simulink model "warplab_siso_unconverted_backup"  (Simulink 6.5)
settings: Solver=ode45  StartTime=0.0  StopTime=30000  RelTol=1e-3
libraries: xbsIndex_r4 x94, WARP_Blockset x4, simulink x1
settings Model: Creator=Melissa.Duarte  LastModifiedBy=cj.steuernagel
settings DebuggingCC: MultiTaskDSMMsg=warning  MultiTaskCondExecSysMsg=none
settings RTWCC: IncludeERTFirstTime=on

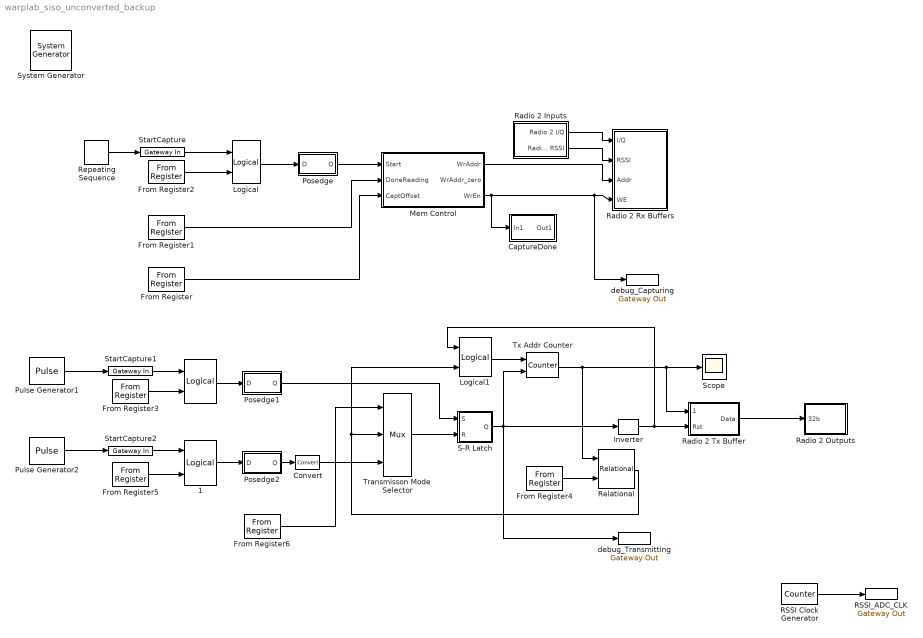
== system warplab_siso_unconverted_backup ==
  " " : xbsIndex_r4/Logical  logical_function=OR  inputs=2  en=off  latency=0  precision=Full  arith_type=Unsigned  n_bits=16  bin_pt=0  align_bp=on  dbl_ovrd=off  block_type=logical
      settings: block_version=9.1.01
  " 1" : xbsIndex_r4/Logical  logical_function=OR  inputs=2  en=off  latency=0  precision=Full  arith_type=Unsigned  n_bits=16  bin_pt=0  align_bp=on  dbl_ovrd=off  block_type=logical
      settings: block_version=9.1.01
  " System Generator" : xbsIndex_r4/ System Generator  Tag=genX  SystemSampleTime=-1  xilinxfamily=Virtex4  part=xc4vsx35  speed=-10  package=ff668  synthesis_tool=XST  directory=./netlist  testbench=off  simulink_period=1  sysclk_period=10  incr_netlist=off  trim_vbits=Everywhere in SubSystem  dbl_ovrd=According to Block Masks  core_generation=According to Block Masks  run_coregen=off  deprecated_control=off  eval_field=0  block_type=sysgen
      settings: block_version=8.2
  CaptureDone : Subsystem
  Convert : xbsIndex_r4/Convert  arith_type=Boolean  n_bits=16  bin_pt=14  quantization=Truncate  overflow=Wrap  latency=0  dbl_ovrd=off  pipeline=off  block_type=convert
  From Register : xbsIndex_r4/From Register  shared_memory_name='CaptOffset'  init=100  period=1  ownership=Locally owned and initialized  arith_type=Unsigned  n_bits=14  bin_pt=0  dbl_ovrd=off  block_type=fromreg
      settings: AttributesFormatString=CaptOffset\n<< %<shared_memory_name> >>  infoedit="Register block that reads data to a shared memory register.  Delay of one sample period."  block_version=8.2
  From Register1 : xbsIndex_r4/From Register  shared_memory_name='DoneReading'  init=0  period=1  ownership=Locally owned and initialized  arith_type=Unsigned  n_bits=1  bin_pt=0  dbl_ovrd=off  block_type=fromreg
      settings: AttributesFormatString=DoneReading\n<< %<shared_memory_name> >>  infoedit="Register block that reads data to a shared memory register.  Delay of one sample period."  block_version=8.2
  From Register2 : xbsIndex_r4/From Register  shared_memory_name='StartCapture'  init=0  period=1  ownership=Locally owned and initialized  arith_type=Unsigned  n_bits=1  bin_pt=0  dbl_ovrd=off  block_type=fromreg
      settings: AttributesFormatString=StartCapture\n<< %<shared_memory_name> >>  infoedit="Register block that reads data to a shared memory register.  Delay of one sample period."  block_version=8.2
  From Register3 : xbsIndex_r4/From Register  shared_memory_name='StartTx'  init=0  period=1  ownership=Locally owned and initialized  arith_type=Unsigned  n_bits=1  bin_pt=0  dbl_ovrd=off  block_type=fromreg
      settings: AttributesFormatString=StartTx\n<< %<shared_memory_name> >>  infoedit="Register block that reads data to a shared memory register.  Delay of one sample period."  block_version=8.2
  From Register4 : xbsIndex_r4/From Register  shared_memory_name='TxLength'  init=2^14-1  period=1  ownership=Locally owned and initialized  arith_type=Unsigned  n_bits=14  bin_pt=0  dbl_ovrd=off  block_type=fromreg
      settings: AttributesFormatString=TxLength\n<< %<shared_memory_name> >>  infoedit="Register block that reads data to a shared memory register.  Delay of one sample period."  block_version=8.2
  From Register5 : xbsIndex_r4/From Register  shared_memory_name='StopTx'  init=0  period=1  ownership=Locally owned and initialized  arith_type=Unsigned  n_bits=1  bin_pt=0  dbl_ovrd=off  block_type=fromreg
      settings: AttributesFormatString=StopTx\n<< %<shared_memory_name> >>  infoedit="Register block that reads data to a shared memory register.  Delay of one sample period."  block_version=8.2
  From Register6 : xbsIndex_r4/From Register  shared_memory_name='TransMode'  init=1  period=1  ownership=Locally owned and initialized  arith_type=Unsigned  n_bits=1  bin_pt=0  dbl_ovrd=off  block_type=fromreg
      settings: AttributesFormatString=TransMode\n<< %<shared_memory_name> >>  infoedit="Register block that reads data to a shared memory register.  Delay of one sample period."  block_version=8.2
  Inverter : xbsIndex_r4/Inverter  en=off  latency=0  dbl_ovrd=off  block_type=inv
      settings: block_version=8.2
  Logical : xbsIndex_r4/Logical  logical_function=OR  inputs=2  en=off  latency=0  precision=Full  arith_type=Unsigned  n_bits=16  bin_pt=0  align_bp=on  dbl_ovrd=off  block_type=logical
      settings: block_version=8.2
  Logical1 : xbsIndex_r4/Logical  logical_function=OR  inputs=2  en=off  latency=0  precision=Full  arith_type=Unsigned  n_bits=16  bin_pt=0  align_bp=on  dbl_ovrd=off  block_type=logical
      settings: block_version=9.1.01
  Mem Control : Subsystem
  Posedge : Subsystem
  Posedge1 : Subsystem
  Posedge2 : Subsystem
  Pulse Generator1 : DiscretePulseGenerator  Period=1000000  PulseWidth=50  PhaseDelay=2
  Pulse Generator2 : DiscretePulseGenerator  Period=1000000  PulseWidth=50  PhaseDelay=20000
  RSSI Clock Generator : xbsIndex_r4/Counter  cnt_type=Free Running  cnt_to=Inf  operation=Up  start_count=0  cnt_by_val=1  arith_type=Unsigned  n_bits=1  bin_pt=0  load_pin=off  rst=off  en=off  explicit_period=on  period=2  dbl_ovrd=off  use_behavioral_HDL=off  use_rpm=off  block_type=counter
      settings: block_version=VER_STRING_GOES_HERE
  RSSI_ADC_CLK : xbsIndex_r4/Gateway Out  hdl_port=on  timing_constraint=None  locs_specified=off  LOCs={}  block_type=gatewayout
      settings: infoedit="Gateway out block.  Converts Xilinx fixed point inputs into ouputs of type Simulink integer, double, or fixed point.<P><P>Hardware notes:  In hardware these blocks become top level output ports or are discarded, depending on how they are configured."  block_version=8.2
  Radio 2 Rx Buffers : Subsystem
  Radio 2 Tx Buffer : Subsystem
  Radio 2 Inputs : Subsystem
  Radio 2 Outputs : Subsystem
  Relational : xbsIndex_r4/Relational  mode=a>=b  en=off  latency=0  dbl_ovrd=off  block_type=relational
      settings: block_version=8.2
  Repeating Sequence : simulink/Sources/Repeating Sequence  SystemSampleTime=-1  rep_seq_t=[1 19999 20000 20001]  rep_seq_y=[0 0 1 0]
  S-R Latch : Subsystem
  Scope : Scope
      settings: YMin=0  YMax=17000  SaveName=ScopeData2
  StartCapture : xbsIndex_r4/Gateway In  arith_type=Unsigned  n_bits=1  bin_pt=0  quantization="Round  (unbiased: +/- Inf)"  overflow=Saturate  period=1  dbl_ovrd=off  timing_constraint=None  locs_specified=off  LOCs={}  block_type=gatewayin
      settings: infoedit="Gateway in block.  Converts inputs of type Simulink integer, double and fixed point to  Xilinx fixed point type.<P><P>Hardware notes:  In hardware these blocks become top level input ports."  block_version=VER_STRING_GOES_HERE
  StartCapture1 : xbsIndex_r4/Gateway In  arith_type=Unsigned  n_bits=1  bin_pt=0  quantization="Round  (unbiased: +/- Inf)"  overflow=Saturate  period=1  dbl_ovrd=off  timing_constraint=None  locs_specified=off  LOCs={}  block_type=gatewayin
      settings: infoedit="Gateway in block.  Converts inputs of type Simulink integer, double and fixed point to  Xilinx fixed point type.<P><P>Hardware notes:  In hardware these blocks become top level input ports."  block_version=VER_STRING_GOES_HERE
  StartCapture2 : xbsIndex_r4/Gateway In  arith_type=Unsigned  n_bits=1  bin_pt=0  quantization="Round  (unbiased: +/- Inf)"  overflow=Saturate  period=1  dbl_ovrd=off  timing_constraint=None  locs_specified=off  LOCs={}  block_type=gatewayin
      settings: infoedit="Gateway in block.  Converts inputs of type Simulink integer, double and fixed point to  Xilinx fixed point type.<P><P>Hardware notes:  In hardware these blocks become top level input ports."  block_version=VER_STRING_GOES_HERE
  Transmisson Mode Selector : xbsIndex_r4/Mux  inputs=2  en=off  latency=0  precision=Full  arith_type=Unsigned  n_bits=16  bin_pt=14  quantization=Truncate  overflow=Wrap  dbl_ovrd=off  block_type=mux
      settings: block_version=9.1.01
  Tx Addr Counter : xbsIndex_r4/Counter  cnt_type=Free Running  cnt_to=Inf  operation=Up  start_count=0  cnt_by_val=1  arith_type=Unsigned  n_bits=14  bin_pt=0  load_pin=off  rst=on  en=on  explicit_period=off  period=1  dbl_ovrd=off  use_behavioral_HDL=off  use_rpm=off  block_type=counter
      settings: block_version=8.2
  debug_Capturing : xbsIndex_r4/Gateway Out  hdl_port=on  timing_constraint=None  locs_specified=off  LOCs={}  block_type=gatewayout
      settings: infoedit="Gateway out block.  Converts Xilinx fixed point inputs into ouputs of type Simulink integer, double, or fixed point.<P><P>Hardware notes:  In hardware these blocks become top level output ports or are discarded, depending on how they are configured."  block_version=8.2
  debug_Transmitting : xbsIndex_r4/Gateway Out  hdl_port=on  timing_constraint=None  locs_specified=off  LOCs={}  block_type=gatewayout
      settings: infoedit="Gateway out block.  Converts Xilinx fixed point inputs into ouputs of type Simulink integer, double, or fixed point.<P><P>Hardware notes:  In hardware these blocks become top level output ports or are discarded, depending on how they are configured."  block_version=8.2
  wires:
  Posedge/1(Q) -> Mem Control/1(Start)
  Mem Control/3(WrEn) -> Radio 2 Rx Buffers/4(WE), debug_Capturing/1, CaptureDone/1(In1)
  Mem Control/1(WrAddr) -> Radio 2 Rx Buffers/3(Addr)
  From Register/1 -> Mem Control/3(CaptOffset)
  From Register1/1 -> Mem Control/2(DoneReading)
  Repeating Sequence/1 -> StartCapture/1
  From Register2/1 -> Logical/2
  Logical/1 -> Posedge/1(D)
  StartCapture/1 -> Logical/1
  Radio 2 Tx Buffer/1(Data) -> Radio 2 Outputs/1(32b)
  Tx Addr Counter/1 -> Relational/1, Radio 2 Tx Buffer/1(RdAddr), Scope/1
  S-R Latch/1(Q) -> Inverter/1, debug_Transmitting/1, Tx Addr Counter/2
  From Register4/1 -> Relational/2
  Inverter/1 -> Radio 2 Tx Buffer/2(Rst), Logical1/1
  Radio 2 Inputs/1(Radio 2 I/Q) -> Radio 2 Rx Buffers/1(I/Q)
  Radio 2 Inputs/2(Radio 2 RSSI) -> Radio 2 Rx Buffers/2(RSSI)
  RSSI Clock Generator/1 -> RSSI_ADC_CLK/1
  Posedge1/1(Q) -> S-R Latch/1(S)
  " "/1 -> Posedge1/1(D)
  From Register3/1 -> " "/2
  StartCapture1/1 -> " "/1
  " 1"/1 -> Posedge2/1(D)
  From Register5/1 -> " 1"/2
  StartCapture2/1 -> " 1"/1
  Relational/1 -> Transmisson Mode Selector/2, Logical1/2
  Logical1/1 -> Tx Addr Counter/1
  From Register6/1 -> Transmisson Mode Selector/1
  Transmisson Mode Selector/1 -> S-R Latch/2(R)
  Pulse Generator2/1 -> StartCapture2/1
  Pulse Generator1/1 -> StartCapture1/1
  Posedge2/1(Q) -> Convert/1
  Convert/1 -> Transmisson Mode Selector/3

== system warplab_siso_unconverted_backup/CaptureDone ==
  In1 : Inport
  Inverter1 : xbsIndex_r4/Inverter  en=off  latency=0  dbl_ovrd=off  block_type=inv
      settings: block_version=8.2
  To Register : xbsIndex_r4/To Register  shared_memory_name='CaptureDone'  init=0  ownership=Locally owned and initialized  explicit_data_type=off  arith_type="Signed  (2's comp)"  n_bits=16  bin_pt=14  dbl_ovrd=off  block_type=toreg
      settings: AttributesFormatString=CaptureDone\n<< %<shared_memory_name> >>  infoedit="Register block that writes data to a shared memory register.  Delay of one sample period."  block_version=8.2
  zero3 : xbsIndex_r4/Constant  arith_type=Boolean  const=1  n_bits=1  bin_pt=0  explicit_period=off  period=1  equ=P=C  opselect=C  inp2=PCIN>>17  opr=+  inp1=P  carry=CIN  dbl_ovrd=off  block_type=constant
      settings: block_version=VER_STRING_GOES_HERE
  Out1 : Outport
  wires:
  zero3/1 -> To Register/2
  Inverter1/1 -> To Register/1
  In1/1 -> Inverter1/1
  To Register/1 -> Out1/1

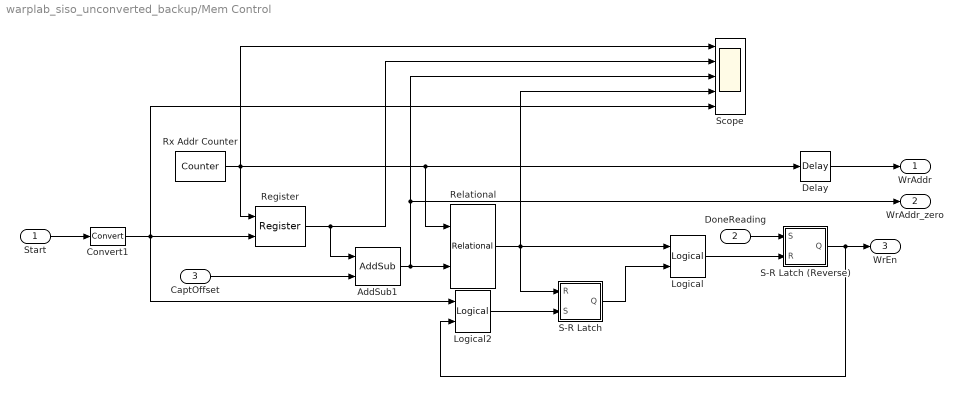
== system warplab_siso_unconverted_backup/Mem Control ==
  Start : Inport
  DoneReading : Inport  Port=2
  CaptOffset : Inport  Port=3
  AddSub1 : xbsIndex_r4/AddSub  mode=Subtraction  use_carryin=off  use_carryout=off  en=off  latency=0  precision=User Defined  arith_type=Unsigned  n_bits=14  bin_pt=0  quantization=Truncate  overflow=Wrap  dbl_ovrd=off  use_behavioral_HDL=off  pipelined=off  use_rpm=on  block_type=addsub
      settings: block_version=8.2
  Convert1 : xbsIndex_r4/Convert  arith_type=Boolean  n_bits=16  bin_pt=14  quantization=Truncate  overflow=Wrap  latency=0  dbl_ovrd=off  pipeline=off  block_type=convert
      settings: block_version=8.2
  Delay : xbsIndex_r4/Delay  en=off  latency=1  dbl_ovrd=off  reg_retiming=off  block_type=delay
      settings: infoedit=Hardware notes: A delay line is a chain, each link of which is an SRL16 followed by a flip-flop. If register retiming is enabled, the delay line is a chain of flip-flops.  block_version=8.2
  Logical : xbsIndex_r4/Logical  logical_function=AND  inputs=2  en=off  latency=0  precision=Full  arith_type=Unsigned  n_bits=16  bin_pt=0  align_bp=on  dbl_ovrd=off  block_type=logical
      settings: block_version=8.2
  Logical2 : xbsIndex_r4/Logical  logical_function=AND  inputs=2  en=off  latency=0  precision=Full  arith_type=Unsigned  n_bits=16  bin_pt=0  align_bp=on  dbl_ovrd=off  block_type=logical
      settings: block_version=8.2
  Register : xbsIndex_r4/Register  init=0  rst=off  en=on  dbl_ovrd=off  block_type=register
      settings: block_version=8.2
  Relational : xbsIndex_r4/Relational  mode=a=b  en=off  latency=0  dbl_ovrd=off  block_type=relational
      settings: block_version=8.2
  Rx Addr Counter : xbsIndex_r4/Counter  cnt_type=Free Running  cnt_to=Inf  operation=Up  start_count=0  cnt_by_val=1  arith_type=Unsigned  n_bits=14  bin_pt=0  load_pin=off  rst=off  en=off  explicit_period=on  period=1  dbl_ovrd=off  use_behavioral_HDL=off  use_rpm=off  block_type=counter
      settings: block_version=8.2
  S-R Latch : Subsystem
  S-R Latch (Reverse) : Subsystem
  Scope : Scope  NumInputPorts=5
      settings: TimeRange=100000  YMin=0~-1~15469.8~0~-1  YMax=17500~1~17098.2~1~1
  WrAddr : Outport
  WrAddr_zero : Outport  Port=2
  WrEn : Outport  Port=3
  wires:
  CaptOffset/1 -> AddSub1/2
  Register/1 -> AddSub1/1, Scope/2
  AddSub1/1 -> Relational/2, Scope/3, WrAddr_zero/1
  DoneReading/1 -> S-R Latch (Reverse)/1(S)
  Relational/1 -> S-R Latch/1(R), Logical/1, Scope/4
  Rx Addr Counter/1 -> Scope/1, Register/1, Delay/1, Relational/1
  Start/1 -> Convert1/1
  S-R Latch (Reverse)/1(Q) -> WrEn/1, Logical2/2
  Delay/1 -> WrAddr/1
  Convert1/1 -> Register/2, Scope/5, Logical2/1
  Logical/1 -> S-R Latch (Reverse)/2(R)
  S-R Latch/1(Q) -> Logical/2
  Logical2/1 -> S-R Latch/2(S)

== system warplab_siso_unconverted_backup/Posedge ==
  D : Inport
  Delay : xbsIndex_r4/Delay  en=off  latency=1  dbl_ovrd=off  reg_retiming=off  block_type=delay
      settings: infoedit=Hardware notes: A delay line is a chain, each link of which is an SRL16 followed by a flip-flop. If register retiming is enabled, the delay line is a chain of flip-flops.  block_version=8.2
  Inverter : xbsIndex_r4/Inverter  en=off  latency=0  dbl_ovrd=off  block_type=inv
      settings: block_version=8.2
  Logical : xbsIndex_r4/Logical  logical_function=AND  inputs=2  en=off  latency=0  precision=Full  arith_type=Unsigned  n_bits=16  bin_pt=0  align_bp=on  dbl_ovrd=off  block_type=logical
      settings: block_version=8.2
  Q : Outport
  wires:
  D/1 -> Inverter/1, Logical/1
  Inverter/1 -> Delay/1
  Delay/1 -> Logical/2
  Logical/1 -> Q/1

== system warplab_siso_unconverted_backup/Posedge1 ==
  D : Inport
  Delay : xbsIndex_r4/Delay  en=off  latency=1  dbl_ovrd=off  reg_retiming=off  block_type=delay
      settings: infoedit=Hardware notes: A delay line is a chain, each link of which is an SRL16 followed by a flip-flop. If register retiming is enabled, the delay line is a chain of flip-flops.  block_version=8.2
  Inverter : xbsIndex_r4/Inverter  en=off  latency=0  dbl_ovrd=off  block_type=inv
      settings: block_version=8.2
  Logical : xbsIndex_r4/Logical  logical_function=AND  inputs=2  en=off  latency=0  precision=Full  arith_type=Unsigned  n_bits=16  bin_pt=0  align_bp=on  dbl_ovrd=off  block_type=logical
      settings: block_version=8.2
  Q : Outport
  wires:
  Logical/1 -> Q/1
  Delay/1 -> Logical/2
  Inverter/1 -> Delay/1
  D/1 -> Logical/1, Inverter/1

== system warplab_siso_unconverted_backup/Posedge2 ==
  D : Inport
  Delay : xbsIndex_r4/Delay  en=off  latency=1  dbl_ovrd=off  reg_retiming=off  block_type=delay
      settings: infoedit=Hardware notes: A delay line is a chain, each link of which is an SRL16 followed by a flip-flop. If register retiming is enabled, the delay line is a chain of flip-flops.  block_version=8.2
  Inverter : xbsIndex_r4/Inverter  en=off  latency=0  dbl_ovrd=off  block_type=inv
      settings: block_version=8.2
  Logical : xbsIndex_r4/Logical  logical_function=AND  inputs=2  en=off  latency=0  precision=Full  arith_type=Unsigned  n_bits=16  bin_pt=0  align_bp=on  dbl_ovrd=off  block_type=logical
      settings: block_version=8.2
  Q : Outport
  wires:
  Logical/1 -> Q/1
  Delay/1 -> Logical/2
  Inverter/1 -> Delay/1
  D/1 -> Logical/1, Inverter/1

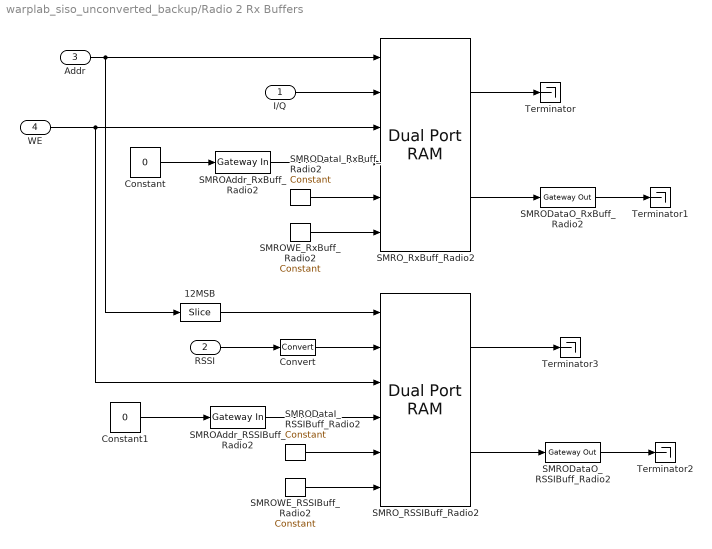
== system warplab_siso_unconverted_backup/Radio 2 Rx Buffers ==
  I/Q : Inport
  RSSI : Inport  Port=2
  Addr : Inport  Port=3
  WE : Inport  Port=4
  12MSB : xbsIndex_r4/Slice  nbits=12  boolean_output=off  mode=Upper Bit Location + Width  bit1=0  base1=MSB of Input  bit0=0  base0=LSB of Input  dbl_ovrd=off  block_type=slice
      settings: infoedit="Extracts a given range of bits from each input sample and presents it at the output.  The output type is ordinarily unsigned with binary point at zero, but can be Boolean when the slice is one bit wide.<P><P>Hardware notes: In hardware this block costs nothing."  block_version=8.2
  Constant : Constant  Value=0  OutDataType=sfix(16)  ConRadixGroup=Use specified scaling  OutScaling=2^0  SampleTime=inf  FramePeriod=inf
  Constant1 : Constant  Value=0  OutDataType=sfix(16)  ConRadixGroup=Use specified scaling  OutScaling=2^0  SampleTime=inf  FramePeriod=inf
  Convert : xbsIndex_r4/Convert  arith_type=Unsigned  n_bits=16  bin_pt=0  quantization=Truncate  overflow=Wrap  latency=0  dbl_ovrd=off  pipeline=off  block_type=convert
      settings: block_version=8.2
  SMROAddr_RSSIBuff_Radio2 : xbsIndex_r4/Gateway In  arith_type=Unsigned  n_bits=11  bin_pt=0  quantization="Round  (unbiased: +/- Inf)"  overflow=Saturate  period=1  dbl_ovrd=off  timing_constraint=None  locs_specified=off  LOCs={}  block_type=gatewayin
      settings: infoedit="Gateway in block.  Converts inputs of type Simulink integer, double and fixed point to  Xilinx fixed point type.<P><P>Hardware notes:  In hardware these blocks become top level input ports."  block_version=VER_STRING_GOES_HERE
  SMROAddr_RxBuff_Radio2 : xbsIndex_r4/Gateway In  arith_type=Unsigned  n_bits=14  bin_pt=0  quantization="Round  (unbiased: +/- Inf)"  overflow=Saturate  period=1  dbl_ovrd=off  timing_constraint=None  locs_specified=off  LOCs={}  block_type=gatewayin
      settings: infoedit="Gateway in block.  Converts inputs of type Simulink integer, double and fixed point to  Xilinx fixed point type.<P><P>Hardware notes:  In hardware these blocks become top level input ports."  block_version=VER_STRING_GOES_HERE
  SMRODataI_RSSIBuff_Radio2 : xbsIndex_r4/Constant  arith_type=Unsigned  const=0  n_bits=32  bin_pt=0  explicit_period=off  period=1  equ=P=C  opselect=C  inp2=PCIN>>17  opr=+  inp1=P  carry=CIN  dbl_ovrd=off  block_type=constant
      settings: block_version=VER_STRING_GOES_HERE
  SMRODataI_RxBuff_Radio2 : xbsIndex_r4/Constant  arith_type=Unsigned  const=0  n_bits=32  bin_pt=0  explicit_period=off  period=1  equ=P=C  opselect=C  inp2=PCIN>>17  opr=+  inp1=P  carry=CIN  dbl_ovrd=off  block_type=constant
      settings: block_version=VER_STRING_GOES_HERE
  SMRODataO_RSSIBuff_Radio2 : xbsIndex_r4/Gateway Out  hdl_port=on  timing_constraint=None  locs_specified=off  LOCs={}  block_type=gatewayout
      settings: infoedit="Gateway out block.  Converts Xilinx fixed point inputs into ouputs of type Simulink integer, double, or fixed point.<P><P>Hardware notes:  In hardware these blocks become top level output ports or are discarded, depending on how they are configured."  xl_area=[0, 0, 0, 0, 0, 0, 0]  block_version=VER_STRING_GOES_HERE
  SMRODataO_RxBuff_Radio2 : xbsIndex_r4/Gateway Out  hdl_port=on  timing_constraint=None  locs_specified=off  LOCs={}  block_type=gatewayout
      settings: infoedit="Gateway out block.  Converts Xilinx fixed point inputs into ouputs of type Simulink integer, double, or fixed point.<P><P>Hardware notes:  In hardware these blocks become top level output ports or are discarded, depending on how they are configured."  xl_area=[0, 0, 0, 0, 0, 0, 0]  block_version=VER_STRING_GOES_HERE
  SMROWE_RSSIBuff_Radio2 : xbsIndex_r4/Constant  arith_type=Boolean  const=0  n_bits=3  bin_pt=0  explicit_period=off  period=1  equ=P=C  opselect=C  inp2=PCIN>>17  opr=+  inp1=P  carry=CIN  dbl_ovrd=off  block_type=constant
      settings: block_version=VER_STRING_GOES_HERE
  SMROWE_RxBuff_Radio2 : xbsIndex_r4/Constant  arith_type=Boolean  const=0  n_bits=3  bin_pt=0  explicit_period=off  period=1  equ=P=C  opselect=C  inp2=PCIN>>17  opr=+  inp1=P  carry=CIN  dbl_ovrd=off  block_type=constant
      settings: block_version=VER_STRING_GOES_HERE
  SMRO_RSSIBuff_Radio2 : xbsIndex_r4/Dual Port RAM  depth=2^12  initVector=1:2^12  distributed_mem=Block RAM  init_a=0  init_b=0  rst_a=off  rst_b=off  en_a=off  en_b=off  latency=1  write_mode_A=Read After Write  write_mode_B=Read After Write  dbl_ovrd=off  optimize=Area  use_rpm=on  block_type=dpram
      settings: block_version=VER_STRING_GOES_HERE
  SMRO_RxBuff_Radio2 : xbsIndex_r4/Dual Port RAM  depth=2^14  initVector=1:2^14  distributed_mem=Block RAM  init_a=0  init_b=0  rst_a=off  rst_b=off  en_a=off  en_b=off  latency=1  write_mode_A=Read After Write  write_mode_B=Read After Write  dbl_ovrd=off  optimize=Area  use_rpm=on  block_type=dpram
      settings: block_version=VER_STRING_GOES_HERE
  Terminator{,1..3} (4 alike) : Terminator
  wires:
  SMRO_RSSIBuff_Radio2/1 -> Terminator3/1
  SMRO_RSSIBuff_Radio2/2 -> SMRODataO_RSSIBuff_Radio2/1
  SMRODataO_RSSIBuff_Radio2/1 -> Terminator2/1
  12MSB/1 -> SMRO_RSSIBuff_Radio2/1
  SMROWE_RSSIBuff_Radio2/1 -> SMRO_RSSIBuff_Radio2/6
  SMRODataI_RSSIBuff_Radio2/1 -> SMRO_RSSIBuff_Radio2/5
  RSSI/1 -> Convert/1
  SMROAddr_RSSIBuff_Radio2/1 -> SMRO_RSSIBuff_Radio2/4
  Constant1/1 -> SMROAddr_RSSIBuff_Radio2/1
  WE/1 -> SMRO_RSSIBuff_Radio2/3, SMRO_RxBuff_Radio2/3
  I/Q/1 -> SMRO_RxBuff_Radio2/2
  Addr/1 -> 12MSB/1, SMRO_RxBuff_Radio2/1
  SMRODataO_RxBuff_Radio2/1 -> Terminator1/1
  SMRO_RxBuff_Radio2/1 -> Terminator/1
  SMROAddr_RxBuff_Radio2/1 -> SMRO_RxBuff_Radio2/4
  SMRO_RxBuff_Radio2/2 -> SMRODataO_RxBuff_Radio2/1
  Constant/1 -> SMROAddr_RxBuff_Radio2/1
  SMRODataI_RxBuff_Radio2/1 -> SMRO_RxBuff_Radio2/5
  SMROWE_RxBuff_Radio2/1 -> SMRO_RxBuff_Radio2/6
  Convert/1 -> SMRO_RSSIBuff_Radio2/2

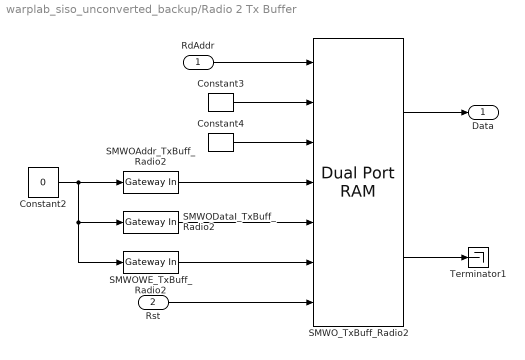
== system warplab_siso_unconverted_backup/Radio 2 Tx Buffer ==
  RdAddr : Inport
  Rst : Inport  Port=2
  Constant2 : Constant  Value=0  OutDataType=sfix(16)  ConRadixGroup=Use specified scaling  OutScaling=2^0  SampleTime=inf  FramePeriod=inf
  Constant3 : xbsIndex_r4/Constant  arith_type=Unsigned  const=0  n_bits=32  bin_pt=0  explicit_period=off  period=1  equ=P=C  opselect=C  inp2=PCIN>>17  opr=+  inp1=P  carry=CIN  dbl_ovrd=off  block_type=constant
      settings: block_version=VER_STRING_GOES_HERE
  Constant4 : xbsIndex_r4/Constant  arith_type=Boolean  const=0  n_bits=1  bin_pt=0  explicit_period=off  period=1  equ=P=C  opselect=C  inp2=PCIN>>17  opr=+  inp1=P  carry=CIN  dbl_ovrd=off  block_type=constant
      settings: block_version=VER_STRING_GOES_HERE
  SMWOAddr_TxBuff_Radio2 : xbsIndex_r4/Gateway In  arith_type=Unsigned  n_bits=14  bin_pt=0  quantization="Round  (unbiased: +/- Inf)"  overflow=Saturate  period=1  dbl_ovrd=off  timing_constraint=None  locs_specified=off  LOCs={}  block_type=gatewayin
      settings: infoedit="Gateway in block.  Converts inputs of type Simulink integer, double and fixed point to  Xilinx fixed point type.<P><P>Hardware notes:  In hardware these blocks become top level input ports."  block_version=VER_STRING_GOES_HERE
  SMWODataI_TxBuff_Radio2 : xbsIndex_r4/Gateway In  arith_type=Unsigned  n_bits=32  bin_pt=0  quantization="Round  (unbiased: +/- Inf)"  overflow=Saturate  period=1  dbl_ovrd=off  timing_constraint=None  locs_specified=off  LOCs={}  block_type=gatewayin
      settings: infoedit="Gateway in block.  Converts inputs of type Simulink integer, double and fixed point to  Xilinx fixed point type.<P><P>Hardware notes:  In hardware these blocks become top level input ports."  block_version=VER_STRING_GOES_HERE
  SMWOWE_TxBuff_Radio2 : xbsIndex_r4/Gateway In  arith_type=Boolean  n_bits=1  bin_pt=0  quantization="Round  (unbiased: +/- Inf)"  overflow=Saturate  period=1  dbl_ovrd=off  timing_constraint=None  locs_specified=off  LOCs={}  block_type=gatewayin
      settings: infoedit="Gateway in block.  Converts inputs of type Simulink integer, double and fixed point to  Xilinx fixed point type.<P><P>Hardware notes:  In hardware these blocks become top level input ports."  block_version=VER_STRING_GOES_HERE
  SMWO_TxBuff_Radio2 : xbsIndex_r4/Dual Port RAM  depth=2^14  initVector=1:2^14  distributed_mem=Block RAM  init_a=0  init_b=0  rst_a=on  rst_b=off  en_a=off  en_b=off  latency=1  write_mode_A=Read After Write  write_mode_B=Read After Write  dbl_ovrd=off  optimize=Area  use_rpm=on  block_type=dpram
      settings: block_version=VER_STRING_GOES_HERE
  Terminator1 : Terminator
  Data : Outport
  wires:
  SMWO_TxBuff_Radio2/2 -> Terminator1/1
  SMWODataI_TxBuff_Radio2/1 -> SMWO_TxBuff_Radio2/5
  SMWOWE_TxBuff_Radio2/1 -> SMWO_TxBuff_Radio2/6
  SMWOAddr_TxBuff_Radio2/1 -> SMWO_TxBuff_Radio2/4
  Constant3/1 -> SMWO_TxBuff_Radio2/2
  Constant4/1 -> SMWO_TxBuff_Radio2/3
  Constant2/1 -> SMWOAddr_TxBuff_Radio2/1, SMWODataI_TxBuff_Radio2/1, SMWOWE_TxBuff_Radio2/1
  RdAddr/1 -> SMWO_TxBuff_Radio2/1
  SMWO_TxBuff_Radio2/1 -> Data/1
  Rst/1 -> SMWO_TxBuff_Radio2/7

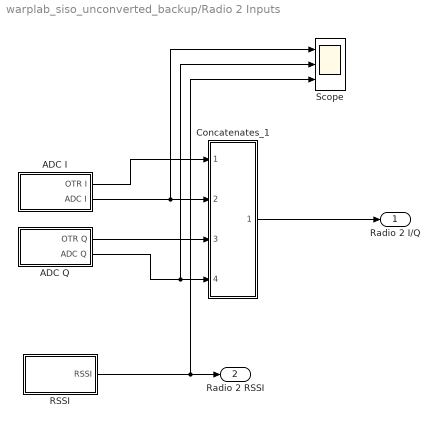
== system warplab_siso_unconverted_backup/Radio 2 Inputs ==
  ADC I : Subsystem
  ADC Q : Subsystem
  Concatenates_1 : Subsystem
  RSSI : Subsystem
  Scope : Scope  NumInputPorts=3
      settings: YMin=-5~-5~-5  YMax=5~5~5
  Radio 2 I/Q : Outport
  Radio 2 RSSI : Outport  Port=2
  wires:
  ADC Q/2(ADC Q) -> Concatenates_1/4(ADC_Q), Scope/2
  ADC Q/1(OTR Q) -> Concatenates_1/3(OTR_Q)
  ADC I/2(ADC I) -> Concatenates_1/2(ADC_I), Scope/1
  ADC I/1(OTR I) -> Concatenates_1/1(OTR_I)
  RSSI/1(RSSI) -> Radio 2 RSSI/1, Scope/3
  Concatenates_1/1(32b) -> Radio 2 I/Q/1

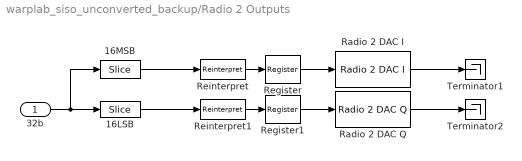
== system warplab_siso_unconverted_backup/Radio 2 Outputs ==
  32b : Inport
  16LSB : xbsIndex_r4/Slice  nbits=16  boolean_output=off  mode=Lower Bit Location + Width  bit1=0  base1=MSB of Input  bit0=0  base0=LSB of Input  dbl_ovrd=off  block_type=slice
      settings: infoedit="Extracts a given range of bits from each input sample and presents it at the output.  The output type is ordinarily unsigned with binary point at zero, but can be Boolean when the slice is one bit wide.<P><P>Hardware notes: In hardware this block costs nothing."  block_version=8.2
  16MSB : xbsIndex_r4/Slice  nbits=16  boolean_output=off  mode=Upper Bit Location + Width  bit1=0  base1=MSB of Input  bit0=0  base0=LSB of Input  dbl_ovrd=off  block_type=slice
      settings: infoedit="Extracts a given range of bits from each input sample and presents it at the output.  The output type is ordinarily unsigned with binary point at zero, but can be Boolean when the slice is one bit wide.<P><P>Hardware notes: In hardware this block costs nothing."  block_version=8.2
  Radio 2 DAC I : WARP_Blockset/WARP Radio ADC//DACs/Radio 2 DAC I  SystemSampleTime=-1
  Radio 2 DAC Q : WARP_Blockset/WARP Radio ADC//DACs/Radio 2 DAC Q  SystemSampleTime=-1
  Register : xbsIndex_r4/Register  init=0  rst=off  en=off  dbl_ovrd=off  block_type=register
      settings: block_version=8.2
  Register1 : xbsIndex_r4/Register  init=0  rst=off  en=off  dbl_ovrd=off  block_type=register
      settings: block_version=8.2
  Reinterpret : xbsIndex_r4/Reinterpret  force_arith_type=on  arith_type="Signed  (2's comp)"  force_bin_pt=on  bin_pt=15  block_type=reinterpret
      settings: infoedit="Changes signal type without altering the binary representation.   You can changed the signal between signed and unsigned, and relocate the binary point.<P><P>Hardware notes: In hardware this block costs nothing.<P><P>Example:  Suppose the input is 6 bits wide, signed, with 2 fractional bits, and the output is forced to unsigned with 0 fractional bits.  Then an input of -2.0 (1110.00 in binary 2's complement) becomes an output of 56 (111000 in binary)."  block_version=8.2
  Reinterpret1 : xbsIndex_r4/Reinterpret  force_arith_type=on  arith_type="Signed  (2's comp)"  force_bin_pt=on  bin_pt=15  block_type=reinterpret
      settings: infoedit="Changes signal type without altering the binary representation.   You can changed the signal between signed and unsigned, and relocate the binary point.<P><P>Hardware notes: In hardware this block costs nothing.<P><P>Example:  Suppose the input is 6 bits wide, signed, with 2 fractional bits, and the output is forced to unsigned with 0 fractional bits.  Then an input of -2.0 (1110.00 in binary 2's complement) becomes an output of 56 (111000 in binary)."  block_version=8.2
  Terminator1 : Terminator
  Terminator2 : Terminator
  wires:
  Radio 2 DAC Q/1 -> Terminator2/1
  Radio 2 DAC I/1 -> Terminator1/1
  Reinterpret1/1 -> Register1/1
  Reinterpret/1 -> Register/1
  16LSB/1 -> Reinterpret1/1
  16MSB/1 -> Reinterpret/1
  32b/1 -> 16LSB/1, 16MSB/1
  Register/1 -> Radio 2 DAC I/1
  Register1/1 -> Radio 2 DAC Q/1

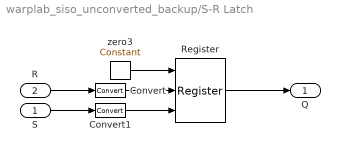
== system warplab_siso_unconverted_backup/S-R Latch ==
  S : Inport
  R : Inport  Port=2
  Convert : xbsIndex_r4/Convert  arith_type=Boolean  n_bits=16  bin_pt=14  quantization=Truncate  overflow=Wrap  latency=0  dbl_ovrd=off  pipeline=off  block_type=convert
      settings: block_version=8.2
  Convert1 : xbsIndex_r4/Convert  arith_type=Boolean  n_bits=16  bin_pt=14  quantization=Truncate  overflow=Wrap  latency=0  dbl_ovrd=off  pipeline=off  block_type=convert
      settings: block_version=8.2
  Register : xbsIndex_r4/Register  init=0  rst=on  en=on  dbl_ovrd=off  block_type=register
      settings: block_version=8.2
  zero3 : xbsIndex_r4/Constant  arith_type=Boolean  const=1  n_bits=1  bin_pt=0  explicit_period=off  period=1  equ=P=C  opselect=C  inp2=PCIN>>17  opr=+  inp1=P  carry=CIN  dbl_ovrd=off  block_type=constant
      settings: block_version=VER_STRING_GOES_HERE
  Q : Outport
  wires:
  Convert1/1 -> Register/3
  Convert/1 -> Register/2
  Register/1 -> Q/1
  S/1 -> Convert1/1
  R/1 -> Convert/1
  zero3/1 -> Register/1

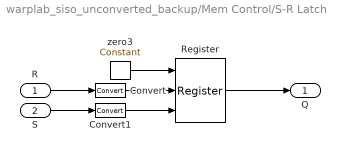
== system warplab_siso_unconverted_backup/Mem Control/S-R Latch ==
  R : Inport
  S : Inport  Port=2
  Convert : xbsIndex_r4/Convert  arith_type=Boolean  n_bits=16  bin_pt=14  quantization=Truncate  overflow=Wrap  latency=0  dbl_ovrd=off  pipeline=off  block_type=convert
      settings: block_version=8.2
  Convert1 : xbsIndex_r4/Convert  arith_type=Boolean  n_bits=16  bin_pt=14  quantization=Truncate  overflow=Wrap  latency=0  dbl_ovrd=off  pipeline=off  block_type=convert
      settings: block_version=8.2
  Register : xbsIndex_r4/Register  init=0  rst=on  en=on  dbl_ovrd=off  block_type=register
      settings: block_version=8.2
  zero3 : xbsIndex_r4/Constant  arith_type=Boolean  const=1  n_bits=1  bin_pt=0  explicit_period=off  period=1  equ=P=C  opselect=C  inp2=PCIN>>17  opr=+  inp1=P  carry=CIN  dbl_ovrd=off  block_type=constant
      settings: block_version=VER_STRING_GOES_HERE
  Q : Outport
  wires:
  Convert1/1 -> Register/3
  Convert/1 -> Register/2
  Register/1 -> Q/1
  S/1 -> Convert1/1
  R/1 -> Convert/1
  zero3/1 -> Register/1

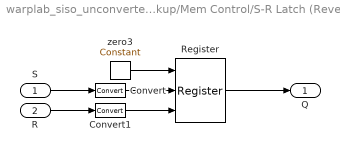
== system warplab_siso_unconverted_backup/Mem Control/S-R Latch (Reverse) ==
  S : Inport
  R : Inport  Port=2
  Convert : xbsIndex_r4/Convert  arith_type=Boolean  n_bits=16  bin_pt=14  quantization=Truncate  overflow=Wrap  latency=0  dbl_ovrd=off  pipeline=off  block_type=convert
      settings: block_version=8.2
  Convert1 : xbsIndex_r4/Convert  arith_type=Boolean  n_bits=16  bin_pt=14  quantization=Truncate  overflow=Wrap  latency=0  dbl_ovrd=off  pipeline=off  block_type=convert
      settings: block_version=8.2
  Register : xbsIndex_r4/Register  init=1  rst=on  en=on  dbl_ovrd=off  block_type=register
      settings: block_version=8.2
  zero3 : xbsIndex_r4/Constant  arith_type=Boolean  const=0  n_bits=1  bin_pt=0  explicit_period=off  period=1  equ=P=C  opselect=C  inp2=PCIN>>17  opr=+  inp1=P  carry=CIN  dbl_ovrd=off  block_type=constant
      settings: block_version=VER_STRING_GOES_HERE
  Q : Outport
  wires:
  zero3/1 -> Register/1
  S/1 -> Convert/1
  R/1 -> Convert1/1
  Register/1 -> Q/1
  Convert/1 -> Register/2
  Convert1/1 -> Register/3

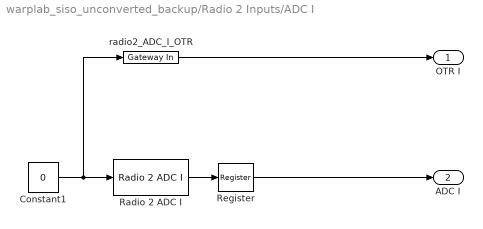
== system warplab_siso_unconverted_backup/Radio 2 Inputs/ADC I ==
  Constant1 : Constant  Value=0  OutDataType=sfix(16)  ConRadixGroup=Use specified scaling  OutScaling=2^0  SampleTime=inf  FramePeriod=inf
  Radio 2 ADC I : WARP_Blockset/WARP Radio ADC//DACs/Radio 2 ADC I  SystemSampleTime=-1  adc_sample_period=1
  Register : xbsIndex_r4/Register  init=0  rst=off  en=off  dbl_ovrd=off  block_type=register
      settings: block_version=8.2
  radio2_ADC_I_OTR : xbsIndex_r4/Gateway In  arith_type=Unsigned  n_bits=1  bin_pt=0  quantization="Round  (unbiased: +/- Inf)"  overflow=Saturate  period=1  dbl_ovrd=off  timing_constraint=None  locs_specified=off  LOCs={}  block_type=gatewayin
      settings: infoedit="Gateway in block.  Converts inputs of type Simulink integer, double and fixed point to  Xilinx fixed point type.<P><P>Hardware notes:  In hardware these blocks become top level input ports."  block_version=VER_STRING_GOES_HERE
  OTR I : Outport
  ADC I : Outport  Port=2
  wires:
  Constant1/1 -> radio2_ADC_I_OTR/1, Radio 2 ADC I/1
  Radio 2 ADC I/1 -> Register/1
  radio2_ADC_I_OTR/1 -> OTR I/1
  Register/1 -> ADC I/1

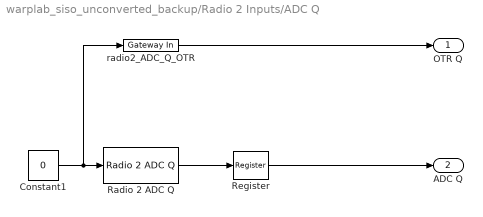
== system warplab_siso_unconverted_backup/Radio 2 Inputs/ADC Q ==
  Constant1 : Constant  Value=0  OutDataType=sfix(16)  ConRadixGroup=Use specified scaling  OutScaling=2^0  SampleTime=inf  FramePeriod=inf
  Radio 2 ADC Q : WARP_Blockset/WARP Radio ADC//DACs/Radio 2 ADC Q  SystemSampleTime=-1  adc_sample_period=1
  Register : xbsIndex_r4/Register  init=0  rst=off  en=off  dbl_ovrd=off  block_type=register
      settings: block_version=8.2
  radio2_ADC_Q_OTR : xbsIndex_r4/Gateway In  arith_type=Unsigned  n_bits=1  bin_pt=0  quantization="Round  (unbiased: +/- Inf)"  overflow=Saturate  period=1  dbl_ovrd=off  timing_constraint=None  locs_specified=off  LOCs={}  block_type=gatewayin
      settings: infoedit="Gateway in block.  Converts inputs of type Simulink integer, double and fixed point to  Xilinx fixed point type.<P><P>Hardware notes:  In hardware these blocks become top level input ports."  block_version=VER_STRING_GOES_HERE
  OTR Q : Outport
  ADC Q : Outport  Port=2
  wires:
  radio2_ADC_Q_OTR/1 -> OTR Q/1
  Radio 2 ADC Q/1 -> Register/1
  Constant1/1 -> radio2_ADC_Q_OTR/1, Radio 2 ADC Q/1
  Register/1 -> ADC Q/1

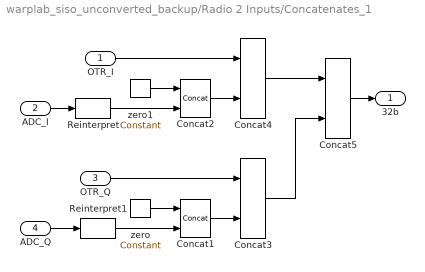
== system warplab_siso_unconverted_backup/Radio 2 Inputs/Concatenates_1 ==
  OTR_I : Inport
  ADC_I : Inport  Port=2
  OTR_Q : Inport  Port=3
  ADC_Q : Inport  Port=4
  Concat{1..5} (5 alike) : xbsIndex_r4/Concat  num_inputs=2  dbl_ovrd=off  block_type=concat
      settings: block_version=8.2
  Reinterpret : xbsIndex_r4/Reinterpret  force_arith_type=on  arith_type=Unsigned  force_bin_pt=on  bin_pt=0  block_type=reinterpret
      settings: infoedit="Changes signal type without altering the binary representation.   You can changed the signal between signed and unsigned, and relocate the binary point.<P><P>Hardware notes: In hardware this block costs nothing.<P><P>Example:  Suppose the input is 6 bits wide, signed, with 2 fractional bits, and the output is forced to unsigned with 0 fractional bits.  Then an input of -2.0 (1110.00 in binary 2's complement) becomes an output of 56 (111000 in binary)."  block_version=8.2
  Reinterpret1 : xbsIndex_r4/Reinterpret  force_arith_type=on  arith_type=Unsigned  force_bin_pt=on  bin_pt=0  block_type=reinterpret
      settings: infoedit="Changes signal type without altering the binary representation.   You can changed the signal between signed and unsigned, and relocate the binary point.<P><P>Hardware notes: In hardware this block costs nothing.<P><P>Example:  Suppose the input is 6 bits wide, signed, with 2 fractional bits, and the output is forced to unsigned with 0 fractional bits.  Then an input of -2.0 (1110.00 in binary 2's complement) becomes an output of 56 (111000 in binary)."  block_version=8.2
  zero : xbsIndex_r4/Constant  arith_type=Unsigned  const=0  n_bits=1  bin_pt=0  explicit_period=off  period=1  equ=P=C  opselect=C  inp2=PCIN>>17  opr=+  inp1=P  carry=CIN  dbl_ovrd=off  block_type=constant
      settings: block_version=VER_STRING_GOES_HERE
  zero1 : xbsIndex_r4/Constant  arith_type=Unsigned  const=0  n_bits=1  bin_pt=0  explicit_period=off  period=1  equ=P=C  opselect=C  inp2=PCIN>>17  opr=+  inp1=P  carry=CIN  dbl_ovrd=off  block_type=constant
      settings: block_version=VER_STRING_GOES_HERE
  32b : Outport
  wires:
  Reinterpret1/1 -> Concat1/2
  Reinterpret/1 -> Concat2/2
  ADC_Q/1 -> Reinterpret1/1
  OTR_Q/1 -> Concat3/1
  ADC_I/1 -> Reinterpret/1
  Concat5/1 -> 32b/1
  OTR_I/1 -> Concat4/1
  Concat3/1 -> Concat5/2
  Concat4/1 -> Concat5/1
  Concat2/1 -> Concat4/2
  zero1/1 -> Concat2/1
  Concat1/1 -> Concat3/2
  zero/1 -> Concat1/1

== system warplab_siso_unconverted_backup/Radio 2 Inputs/RSSI ==
  Constant1 : Constant  Value=0  OutDataType=sfix(16)  ConRadixGroup=Use specified scaling  OutScaling=2^0  SampleTime=inf  FramePeriod=inf
  radio2_RSSI : xbsIndex_r4/Gateway In  arith_type=Unsigned  n_bits=10  bin_pt=0  quantization=Truncate  overflow=Wrap  period=4  dbl_ovrd=off  timing_constraint=None  locs_specified=off  LOCs={}  block_type=gatewayin
      settings: infoedit="Gateway in block.  Converts inputs of type Simulink integer, double and fixed point to  Xilinx fixed point type.<P><P>Hardware notes:  In hardware these blocks become top level input ports."  block_version=VER_STRING_GOES_HERE
  RSSI : Outport
  wires:
  Constant1/1 -> radio2_RSSI/1
  radio2_RSSI/1 -> RSSI/1
